simulink model "Hop"  (R2020b)
settings: Solver=VariableStepAuto  StartTime=0.0  StopTime=125  FixedStep=0.01  RelTol=1e-3
undefined symbols (not defined in the file): A, Cd, flux, g, M0, Mfuel0, rho, Vexaust
libraries: simulink x5, vrlib x4, pid_lib x3
settings Model: NumberOfSteps=1000  EnablePacing=on  PacingRate=1.300000  VariantFading=off  Creator=65171  LastModifiedBy=65171
settings ConfigComp: PSAutoStubLUT=on

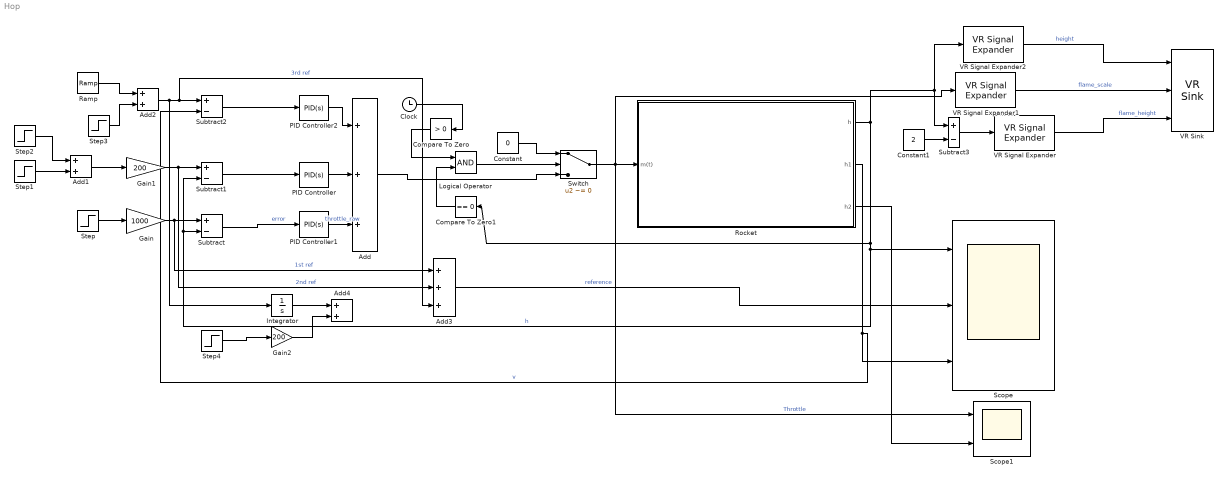
== system Hop ==
  Add : Sum  Inputs=+++
  Add1 : Sum
  Add2 : Sum
  Add3 : Sum  Inputs=+++
  Add4 : Sum
  Clock : Clock
  Compare To Zero : simulink/Logic and Bit Operations/Compare To Zero  relop=>  OutDataTypeStr=boolean
  Compare To Zero1 : simulink/Logic and Bit Operations/Compare To Zero  relop===  OutDataTypeStr=boolean
  Constant : Constant  Value=0
  Constant1 : Constant  Value=2
  Gain : Gain  Gain=1000
  Gain1 : Gain  Gain=200
  Gain2 : Gain  Gain=200
  Integrator : Integrator
  Logical Operator : Logic  AllPortsSameDT=off  OutDataTypeStr=boolean
  PID Controller : pid_lib/PID Controller  Controller=PID  Form=Parallel  TimeDomain=Continuous-time  UseExternalTs=off  SampleTime=-1  IntegratorMethod=Forward Euler  FilterMethod=Forward Euler  ControllerParametersSource=internal  P=0.18  I=0.000000002  D=0.55  UseFilter=on  N=100  TunerSelectOption=Transfer Function Based (PID Tuner App)  InitialConditionSource=internal  InitialConditionForIntegrator=0  InitialConditionForFilter=0  DifferentiatorICPrevScaledInput=0  ExternalReset=none  TrackingMode=off  Kt=1  LimitOutput=on  SatLimitsSource=internal  UpperSaturationLimit=1  LowerSaturationLimit=0.1  LinearizeAsGain=on  AntiWindupMode=none  Kb=1  POutMin=[]  POutMax=[]  IOutMin=[]  IOutMax=[]  DOutMin=[]  DOutMax=[]  NOutMin=[]  NOutMax=[]  SumOutMin=[]  SumOutMax=[]  SaturationOutMin=[]  SaturationOutMax=[]  PParamMin=[]  PParamMax=[]  IParamMin=[]  IParamMax=[]  DParamMin=[]  DParamMax=[]  NParamMin=[]  NParamMax=[]  KbParamMin=[]  KbParamMax=[]  KtParamMin=[]  KtParamMax=[]  KbOutMin=[]  KbOutMax=[]  KtOutMin=[]  KtOutMax=[]  IntegratorOutMin=[]  IntegratorOutMax=[]  FilterOutMin=[]  FilterOutMax=[]  SumI1OutMin=[]  SumI1OutMax=[]  SumI2OutMin=[]  SumI2OutMax=[]  SumI3OutMin=[]  SumI3OutMax=[]  SumI4OutMin=[]  SumI4OutMax=[]  SumDOutMin=[]  SumDOutMax=[]  DifferentiatorOutMin=[]  DifferentiatorOutMax=[]  FilterDiffOutCoefMin=[]  FilterDiffOutCoefMax=[]  ReciprocalOutMin=[]  ReciprocalOutMax=[]  SumDenOutMin=[]  SumDenOutMax=[]  SumNumOutMin=[]  SumNumOutMax=[]  DivideOutMin=[]  DivideOutMax=[]  UdiffTsProdOutMin=[]  UdiffTsProdOutMax=[]  NTsProdOutMin=[]  NTsProdOutMax=[]  UintegralTsProdOutMin=[]  UintegralTsProdOutMax=[]  UngainTsProdOutMin=[]  UngainTsProdOutMax=[]  IntegratorContinuousStateAttributes=''  IntegratorStateMustResolveToSignalObject=off  IntegratorRTWStateStorageClass=Auto  FilterContinuousStateAttributes=''  FilterStateMustResolveToSignalObject=off  FilterRTWStateStorageClass=Auto  ParallelPVariant=InternalParameters  IdealPVariant=Disabled  IVariant=InternalParameters  DVariant=InternalParameters  IntegratorVariant=Continuous  SatVariant=Enabled  AWVariant=Passthrough  PCopyVariant=Disabled  TRVariant=Disabled  FdbkBlocksVariant=Forward  IdealPFdbkVariant=Disabled  SatFdbkVariant=Disabled  DerivativeFilterVariant=ContFilter  NVariant=InternalParameters  NCopyVariant=Disabled  FilterICVariant=InternalICsFilter  IntegratorICVariant=InternalICs  ExternalResetVariant=Disabled  TRSumVariant=Passthrough  SumFdbkVariant=Disabled  SumVariant=Sum_PID  TsampFilterVariant=InternalTs  TsampNgainVariant=Passthrough  TsampIntegralVariant=Passthrough  ExternalSaturationOutDataTypeStr=Inherit: Same as second input
  PID Controller1 : pid_lib/PID Controller  Controller=PID  Form=Parallel  TimeDomain=Continuous-time  UseExternalTs=off  SampleTime=0.01  IntegratorMethod=Forward Euler  FilterMethod=Forward Euler  ControllerParametersSource=internal  P=0.039  I=0.00003  D=0.2  UseFilter=on  N=100  TunerSelectOption=Transfer Function Based (PID Tuner App)  InitialConditionSource=internal  InitialConditionForIntegrator=0  InitialConditionForFilter=0  DifferentiatorICPrevScaledInput=0  ExternalReset=none  TrackingMode=off  Kt=1  LimitOutput=on  SatLimitsSource=internal  UpperSaturationLimit=1  LowerSaturationLimit=0.1  LinearizeAsGain=on  AntiWindupMode=none  Kb=1  POutMin=[]  POutMax=[]  IOutMin=[]  IOutMax=[]  DOutMin=[]  DOutMax=[]  NOutMin=[]  NOutMax=[]  SumOutMin=[]  SumOutMax=[]  SaturationOutMin=[]  SaturationOutMax=[]  PParamMin=[]  PParamMax=[]  IParamMin=[]  IParamMax=[]  DParamMin=[]  DParamMax=[]  NParamMin=[]  NParamMax=[]  KbParamMin=[]  KbParamMax=[]  KtParamMin=[]  KtParamMax=[]  KbOutMin=[]  KbOutMax=[]  KtOutMin=[]  KtOutMax=[]  IntegratorOutMin=[]  IntegratorOutMax=[]  FilterOutMin=[]  FilterOutMax=[]  SumI1OutMin=[]  SumI1OutMax=[]  SumI2OutMin=[]  SumI2OutMax=[]  SumI3OutMin=[]  SumI3OutMax=[]  SumI4OutMin=[]  SumI4OutMax=[]  SumDOutMin=[]  SumDOutMax=[]  DifferentiatorOutMin=[]  DifferentiatorOutMax=[]  FilterDiffOutCoefMin=[]  FilterDiffOutCoefMax=[]  ReciprocalOutMin=[]  ReciprocalOutMax=[]  SumDenOutMin=[]  SumDenOutMax=[]  SumNumOutMin=[]  SumNumOutMax=[]  DivideOutMin=[]  DivideOutMax=[]  UdiffTsProdOutMin=[]  UdiffTsProdOutMax=[]  NTsProdOutMin=[]  NTsProdOutMax=[]  UintegralTsProdOutMin=[]  UintegralTsProdOutMax=[]  UngainTsProdOutMin=[]  UngainTsProdOutMax=[]  IntegratorContinuousStateAttributes=''  IntegratorStateMustResolveToSignalObject=off  IntegratorRTWStateStorageClass=Auto  FilterContinuousStateAttributes=''  FilterStateMustResolveToSignalObject=off  FilterRTWStateStorageClass=Auto  ParallelPVariant=InternalParameters  IdealPVariant=Disabled  IVariant=InternalParameters  DVariant=InternalParameters  IntegratorVariant=Continuous  SatVariant=Enabled  AWVariant=Passthrough  PCopyVariant=Disabled  TRVariant=Disabled  FdbkBlocksVariant=Forward  IdealPFdbkVariant=Disabled  SatFdbkVariant=Disabled  DerivativeFilterVariant=ContFilter  NVariant=InternalParameters  NCopyVariant=Disabled  FilterICVariant=InternalICsFilter  IntegratorICVariant=InternalICs  ExternalResetVariant=Disabled  TRSumVariant=Passthrough  SumFdbkVariant=Disabled  SumVariant=Sum_PID  TsampFilterVariant=InternalTs  TsampNgainVariant=Passthrough  TsampIntegralVariant=Passthrough  ExternalSaturationOutDataTypeStr=Inherit: Same as second input
  PID Controller2 : pid_lib/PID Controller  Controller=PID  Form=Parallel  TimeDomain=Continuous-time  UseExternalTs=off  SampleTime=-1  IntegratorMethod=Forward Euler  FilterMethod=Forward Euler  ControllerParametersSource=internal  P=0.0412036276592499  I=0.00338411296359241  D=-0.0265583864380634  UseFilter=on  N=1.55143565499887  TunerSelectOption=Transfer Function Based (PID Tuner App)  InitialConditionSource=internal  InitialConditionForIntegrator=0  InitialConditionForFilter=0  DifferentiatorICPrevScaledInput=0  ExternalReset=none  TrackingMode=off  Kt=1  LimitOutput=on  SatLimitsSource=internal  UpperSaturationLimit=1  LowerSaturationLimit=0.1  LinearizeAsGain=on  AntiWindupMode=none  Kb=1  POutMin=[]  POutMax=[]  IOutMin=[]  IOutMax=[]  DOutMin=[]  DOutMax=[]  NOutMin=[]  NOutMax=[]  SumOutMin=[]  SumOutMax=[]  SaturationOutMin=[]  SaturationOutMax=[]  PParamMin=[]  PParamMax=[]  IParamMin=[]  IParamMax=[]  DParamMin=[]  DParamMax=[]  NParamMin=[]  NParamMax=[]  KbParamMin=[]  KbParamMax=[]  KtParamMin=[]  KtParamMax=[]  KbOutMin=[]  KbOutMax=[]  KtOutMin=[]  KtOutMax=[]  IntegratorOutMin=[]  IntegratorOutMax=[]  FilterOutMin=[]  FilterOutMax=[]  SumI1OutMin=[]  SumI1OutMax=[]  SumI2OutMin=[]  SumI2OutMax=[]  SumI3OutMin=[]  SumI3OutMax=[]  SumI4OutMin=[]  SumI4OutMax=[]  SumDOutMin=[]  SumDOutMax=[]  DifferentiatorOutMin=[]  DifferentiatorOutMax=[]  FilterDiffOutCoefMin=[]  FilterDiffOutCoefMax=[]  ReciprocalOutMin=[]  ReciprocalOutMax=[]  SumDenOutMin=[]  SumDenOutMax=[]  SumNumOutMin=[]  SumNumOutMax=[]  DivideOutMin=[]  DivideOutMax=[]  UdiffTsProdOutMin=[]  UdiffTsProdOutMax=[]  NTsProdOutMin=[]  NTsProdOutMax=[]  UintegralTsProdOutMin=[]  UintegralTsProdOutMax=[]  UngainTsProdOutMin=[]  UngainTsProdOutMax=[]  IntegratorContinuousStateAttributes=''  IntegratorStateMustResolveToSignalObject=off  IntegratorRTWStateStorageClass=Auto  FilterContinuousStateAttributes=''  FilterStateMustResolveToSignalObject=off  FilterRTWStateStorageClass=Auto  ParallelPVariant=InternalParameters  IdealPVariant=Disabled  IVariant=InternalParameters  DVariant=InternalParameters  IntegratorVariant=Continuous  SatVariant=Enabled  AWVariant=Passthrough  PCopyVariant=Disabled  TRVariant=Disabled  FdbkBlocksVariant=Forward  IdealPFdbkVariant=Disabled  SatFdbkVariant=Disabled  DerivativeFilterVariant=ContFilter  NVariant=InternalParameters  NCopyVariant=Disabled  FilterICVariant=InternalICsFilter  IntegratorICVariant=InternalICs  ExternalResetVariant=Disabled  TRSumVariant=Passthrough  SumFdbkVariant=Disabled  SumVariant=Sum_PID  TsampFilterVariant=InternalTs  TsampNgainVariant=Passthrough  TsampIntegralVariant=Passthrough  ExternalSaturationOutDataTypeStr=Inherit: Same as second input
  Ramp : simulink/Sources/Ramp  slope=0.8  start=100  InitialOutput=0
  Rocket : Subsystem
  Scope : Scope  NumInputPorts=3
  Scope1 : Scope  NumInputPorts=2
  Step : Step  Time=70  Before=1  After=0  SampleTime=0.01
  Step1 : Step  Time=70  SampleTime=0.01
  Step2 : Step  Time=100  After=-1  SampleTime=0.01
  Step3 : Step  Time=100  After=-20  SampleTime=0.01
  Step4 : Step  Time=100  SampleTime=0.01
  Subtract{,1..3} (4 alike) : Sum  Inputs=+-
  Switch : Switch  Criteria=u2 ~= 0
  VR Signal Expander : vrlib/VR Signal Expander  outwidth=3  outidx=2
  VR Signal Expander1 : vrlib/VR Signal Expander  outwidth=3  outidx=2
  VR Signal Expander2 : vrlib/VR Signal Expander  outwidth=3  outidx=2
  VR Sink : vrlib/VR Sink  InstantiateOnLoad=on  SampleTime=0.1  ViewEnable=on  RemoteChange=off  RemoteView=off  FieldsWritten=sn_Transform.translation.3.1.1.double#Flame.scale.3.1.1.double#Flame.translation.3.1.1.double  WorldFileName=3dworld.x3d  WorldDescription=Hopper  AutoView=on  VideoDimensions=[]  AllowVariableSize=off
  wires:
  Subtract/1 -> PID Controller1/1  "error"
  Rocket/2(h1) -> Scope/3, Subtract2/2  "v"
  Rocket/1(h) -> Subtract1/2, Subtract/2, Scope/1, Compare To Zero1/1, VR Signal Expander2/1, Subtract3/1  "h"
  Step/1 -> Gain/1
  Gain/1 -> Add3/1, Subtract/1  "1st ref"
  Gain1/1 -> Add3/2, Subtract1/1  "2nd ref"
  Subtract1/1 -> PID Controller/1
  Add/1 -> Switch/3
  Ramp/1 -> Add2/1
  Add1/1 -> Gain1/1
  Step1/1 -> Add1/2
  Step2/1 -> Add1/1
  PID Controller1/1 -> Add/3  "throttle_raw"
  Subtract2/1 -> PID Controller2/1
  Step3/1 -> Add2/2
  Logical Operator/1 -> Switch/2
  Clock/1 -> Compare To Zero/1
  Compare To Zero/1 -> Logical Operator/1
  Compare To Zero1/1 -> Logical Operator/2
  Constant/1 -> Switch/1
  Switch/1 -> Scope1/1, VR Signal Expander1/1, Rocket/1(m(t))  "Throttle"
  VR Signal Expander1/1 -> VR Sink/2  "flame_scale"
  Constant1/1 -> Subtract3/2
  VR Signal Expander2/1 -> VR Sink/1  "height"
  Subtract3/1 -> VR Signal Expander/1
  VR Signal Expander/1 -> VR Sink/3  "flame_height"
  Add2/1 -> Integrator/1, Add3/3, Subtract2/1  "3rd ref"
  Add3/1 -> Scope/2  "reference"
  Integrator/1 -> Add4/1
  Gain2/1 -> Add4/2
  Step4/1 -> Gain2/1
  Rocket/3(h2) -> Scope1/2
  PID Controller/1 -> Add/2
  PID Controller2/1 -> Add/1

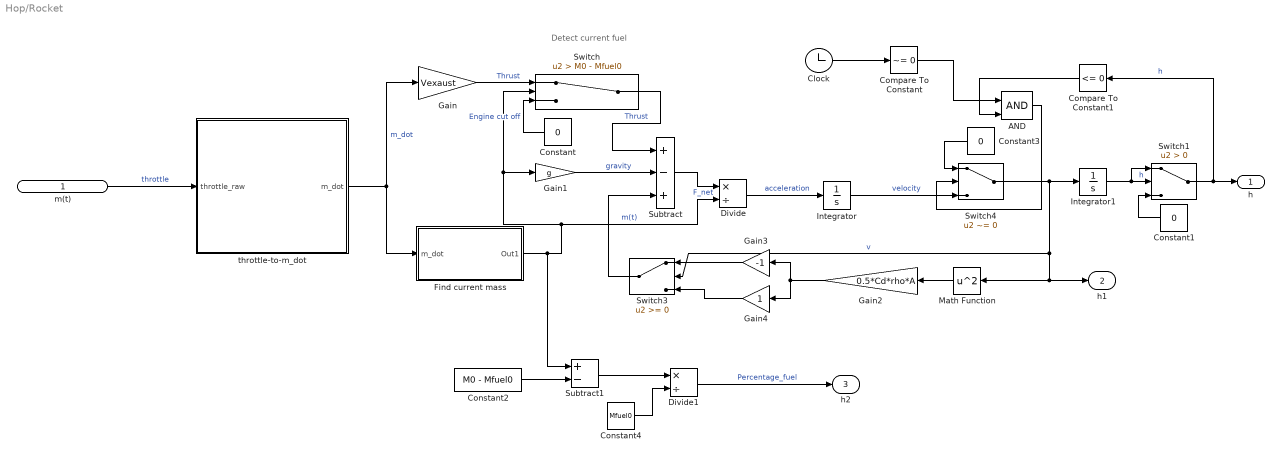
== system Hop/Rocket ==
  note: Detect current fuel
  m(t) : Inport
  AND : Logic  IconShape=distinctive  AllPortsSameDT=off  OutDataTypeStr=boolean
  Clock : Clock
  Compare To Constant : simulink/Logic and Bit Operations/Compare To Constant  relop=~=  const=0  OutDataTypeStr=boolean
  Compare To Constant1 : simulink/Logic and Bit Operations/Compare To Constant  relop=<=  const=0  OutDataTypeStr=boolean
  Constant : Constant  Value=0
  Constant1 : Constant  Value=0
  Constant2 : Constant  Value=M0 - Mfuel0
  Constant3 : Constant  Value=0
  Constant4 : Constant  Value=Mfuel0
  Divide : Product  Inputs=*/
  Divide1 : Product  Inputs=*/
  Find current mass : Subsystem
  Gain : Gain  Gain=Vexaust
  Gain1 : Gain  Gain=g
  Gain2 : Gain  Gain=0.5*Cd*rho*A
  Gain3 : Gain  Gain=-1
  Gain4 : Gain
  Integrator : Integrator  ContinuousStateAttributes='velocity'
  Integrator1 : Integrator  ContinuousStateAttributes='height'
  Math Function : Math  Operator=square  OutDataTypeStr=double  SaturateOnIntegerOverflow=on
  Subtract : Sum  Inputs=+-+
  Subtract1 : Sum  Inputs=+-
  Switch : Switch  Criteria=u2 > Threshold  Threshold=M0 - Mfuel0
  Switch1 : Switch  Criteria=u2 > Threshold
  Switch3 : Switch
  Switch4 : Switch  Criteria=u2 ~= 0
  throttle-to-m_dot : Subsystem
  h : Outport
  h1 : Outport  Port=2
  h2 : Outport  Port=3
  wires:
  Gain/1 -> Switch/1  "Thrust"
  Subtract/1 -> Divide/1  "F_net"
  Integrator1/1 -> Switch1/1, Switch1/2  "h"
  Find current mass/1(Out1) -> Subtract1/1, Switch/2, Gain1/1, Divide/2  "m(t)"
  m(t)/1 -> throttle-to-m_dot/1(throttle_raw)  "throttle"
  throttle-to-m_dot/1(m_dot) -> Gain/1, Find current mass/1(m_dot)  "m_dot"
  Switch/1 -> Subtract/1  "Thrust"
  Constant/1 -> Switch/3  "Engine cut off"
  Switch1/1 -> Compare To Constant1/1, h/1  "h"
  Constant1/1 -> Switch1/3
  Math Function/1 -> Gain2/1
  Gain1/1 -> Subtract/2  "gravity"
  Gain3/1 -> Switch3/1
  Gain4/1 -> Switch3/3
  Gain2/1 -> Gain4/1, Gain3/1
  Switch3/1 -> Subtract/3
  Switch4/1 -> Integrator1/1, Switch3/2, h1/1, Math Function/1  "v"
  Divide/1 -> Integrator/1  "acceleration"
  Clock/1 -> Compare To Constant/1
  Compare To Constant/1 -> AND/1
  Compare To Constant1/1 -> AND/2
  AND/1 -> Switch4/2
  Constant3/1 -> Switch4/1
  Integrator/1 -> Switch4/3  "velocity"
  Constant2/1 -> Subtract1/2
  Subtract1/1 -> Divide1/1
  Constant4/1 -> Divide1/2
  Divide1/1 -> h2/1  "Percentage_fuel"

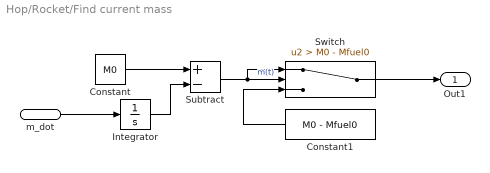
== system Hop/Rocket/Find current mass ==
  m_dot : Inport
  Constant : Constant  Value=M0
  Constant1 : Constant  Value=M0 - Mfuel0
  Integrator : Integrator  ContinuousStateAttributes='deltam'
  Subtract : Sum  Inputs=+-
  Switch : Switch  Criteria=u2 > Threshold  Threshold=M0 - Mfuel0
  Out1 : Outport
  wires:
  Constant/1 -> Subtract/1
  m_dot/1 -> Integrator/1
  Integrator/1 -> Subtract/2
  Subtract/1 -> Switch/1, Switch/2  "m(t)"
  Switch/1 -> Out1/1
  Constant1/1 -> Switch/3

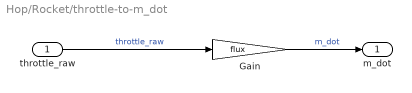
== system Hop/Rocket/throttle-to-m_dot ==
  throttle_raw : Inport
  Gain : Gain  Gain=flux
  m_dot : Outport
  wires:
  Gain/1 -> m_dot/1  "m_dot"
  throttle_raw/1 -> Gain/1  "throttle_raw"
